simulink model "BEV_Laengsdynamikmodell_v2"  (R2024a)
settings: configuration reference "SharedConfig" (kept outside this file)
values from neighbouring files (symbols this model uses):
  acc_cycle_flag = 0    [simulink_function_handle_v2.m]
  battery = sim_BTMS_interface(battery,config_battery, config_vehicle)    [init_simulation.m]    (also in simulink_function_handle_v2.m = evalin('base', 'battery'))
  config_battery = read_json_config("config/conf_battery.json")    [Sim_v2.m]    (also in init_simulation.m = evalin('base', 'config_battery'); simulink_function_handle_v2.m = cell_loader(config_battery, bat_cell_capacity, bat_celltype )
  config_gearbox = evalin("base", "config_gearbox")    [simulink_function_handle_v2.m]
  config_Inverter = read_json_config("config/conf_Inverter.json")    [Sim_v2.m]
  config_motor = evalin("base","config_motor")    [simulink_function_handle_v2.m]
  config_vehicle = read_json_config(vehicle_config_file)    [Sim_v2.m]    (also in import_dc_cycle.m = evalin('base', 'config_vehicle'); init_simulation.m = evalin('base', 'config_vehicle'); simulink_function_handle_v2.m = evalin('base','config_vehicle'))
  k_FW = 410/(14e3)^2.5    (= 1.76792471652e-08)    [simulink_function_handle_v2.m]
  ModuleType1 = evalin("base","ModuleType1")    [simulink_function_handle_v2.m]
undefined symbols (not defined in the file or in its folder): Analyse, battery_builder_rtmsupport, GB, gcbh, gearbox_map, ModuleAssembly1, motormap
libraries: spsParallelRLCBranchLib x20, nesl_utility x18, GD_Batterymodel_NSGAII_1_lib x12, BatteryProtection x9, spsControlledCurrentSourceLib x8, spsVoltageMeasurementLib x8, fl_lib x7, dspstat3 x4, spsDCVoltageSourceLib x4, spspowerguiLib x4, simulink x3, eePmsmCurrentReferenceGen x2
(part 4 of 5)

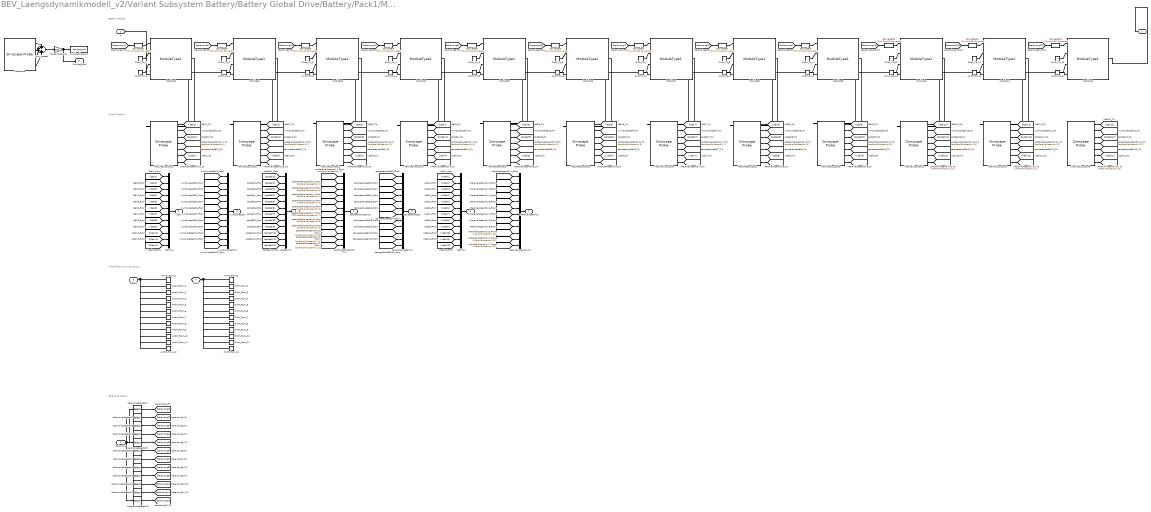
== system BEV_Laengsdynamikmodell_v2/Variant Subsystem Battery/Battery Global Drive/Battery/Pack1/ModuleAssembly1 ==
  note: Battery Modules
  note: Output Signals
  note: Thermal Boundary Conditions
  note: Balancing Signals
  balancing : Inport  PortDimensions=120
  AmbH_From_1 : ConnectionLabel  Label=ambH_1
  AmbH_From_10 : ConnectionLabel  Label=ambH_10
  AmbH_From_11 : ConnectionLabel  Label=ambH_11
  AmbH_From_12 : ConnectionLabel  Label=ambH_12
  AmbH_From_2 : ConnectionLabel  Label=ambH_2
  AmbH_From_3 : ConnectionLabel  Label=ambH_3
  AmbH_From_4 : ConnectionLabel  Label=ambH_4
  AmbH_From_5 : ConnectionLabel  Label=ambH_5
  AmbH_From_6 : ConnectionLabel  Label=ambH_6
  AmbH_From_7 : ConnectionLabel  Label=ambH_7
  AmbH_From_8 : ConnectionLabel  Label=ambH_8
  AmbH_From_9 : ConnectionLabel  Label=ambH_9
  AmbH_To_1 : ConnectionLabel  Label=ambH_1
  AmbH_To_10 : ConnectionLabel  Label=ambH_10
  AmbH_To_11 : ConnectionLabel  Label=ambH_11
  AmbH_To_12 : ConnectionLabel  Label=ambH_12
  AmbH_To_2 : ConnectionLabel  Label=ambH_2
  AmbH_To_3 : ConnectionLabel  Label=ambH_3
  AmbH_To_4 : ConnectionLabel  Label=ambH_4
  AmbH_To_5 : ConnectionLabel  Label=ambH_5
  AmbH_To_6 : ConnectionLabel  Label=ambH_6
  AmbH_To_7 : ConnectionLabel  Label=ambH_7
  AmbH_To_8 : ConnectionLabel  Label=ambH_8
  AmbH_To_9 : ConnectionLabel  Label=ambH_9
  ClntH_From_1 : ConnectionLabel  Label=clntH_1
  ClntH_From_10 : ConnectionLabel  Label=clntH_10
  ClntH_From_11 : ConnectionLabel  Label=clntH_11
  ClntH_From_12 : ConnectionLabel  Label=clntH_12
  ClntH_From_2 : ConnectionLabel  Label=clntH_2
  ClntH_From_3 : ConnectionLabel  Label=clntH_3
  ClntH_From_4 : ConnectionLabel  Label=clntH_4
  ClntH_From_5 : ConnectionLabel  Label=clntH_5
  ClntH_From_6 : ConnectionLabel  Label=clntH_6
  ClntH_From_7 : ConnectionLabel  Label=clntH_7
  ClntH_From_8 : ConnectionLabel  Label=clntH_8
  ClntH_From_9 : ConnectionLabel  Label=clntH_9
  ClntH_To_1 : ConnectionLabel  Label=clntH_1
  ClntH_To_10 : ConnectionLabel  Label=clntH_10
  ClntH_To_11 : ConnectionLabel  Label=clntH_11
  ClntH_To_12 : ConnectionLabel  Label=clntH_12
  ClntH_To_2 : ConnectionLabel  Label=clntH_2
  ClntH_To_3 : ConnectionLabel  Label=clntH_3
  ClntH_To_4 : ConnectionLabel  Label=clntH_4
  ClntH_To_5 : ConnectionLabel  Label=clntH_5
  ClntH_To_6 : ConnectionLabel  Label=clntH_6
  ClntH_To_7 : ConnectionLabel  Label=clntH_7
  ClntH_To_8 : ConnectionLabel  Label=clntH_8
  ClntH_To_9 : ConnectionLabel  Label=clntH_9
  Converter{1..12} (12 alike) : nesl_utility/Simulink-PS Converter  PhysicalDomain=network_engine_domain  SubClassName=ps_input  LeftPortType=input  RightPortType=output  PseudoPeriodic=off  Frequencies=[]  NoiseDistribution=none  NoiseParameters=[]  Unit=1  AffineConversion=off  FilteringAndDerivatives=provide  SimscapeFilterOrder=1  InputFilterTimeConstant=0.001  UdotUserProvided=0
  LossProbe : SimscapeProbe  BoundBlock=59725  Variables={Cell1.power_dissipated, CoolantResistor.Q, balancingResistor.power_dissipated, balancingSwitch.power_dissipated}
  Module01 : GD_Batterymodel_NSGAII_1_lib/Modules/ModuleType1  SOC_vecCell=ModuleType1.SOC_vecCell  T_vecCell=ModuleType1.T_vecCell K  V0_matCell=ModuleType1.V0_matCell V  V_rangeCell=ModuleType1.V_rangeCell V  R0_matCell=ModuleType1.R0_matCell Ohm  AHCell=ModuleType1.AHCell A*hr  extrapolation_optionCell=simscape.enum.extrapolation.nearest  R1_matCell=ModuleType1.R1_matCell Ohm  tau1_matCell=ModuleType1.tau1_matCell s  R2_matCell=ModuleType1.R2_matCell Ohm  tau2_matCell=ModuleType1.tau2_matCell s  thermal_massCell=ModuleType1.thermal_massCell J/K  CoolantResistance=ModuleType1.CoolantResistance K/W  AmbientResistance=ModuleType1.AmbientResistance K/W  CellBalancingClosedResistance=ModuleType1.CellBalancingClosedResistance Ohm  CellBalancingOpenConductance=ModuleType1.CellBalancingOpenConductance 1/Ohm  CellBalancingThreshold=ModuleType1.CellBalancingThreshold  CellBalancingResistance=ModuleType1.CellBalancingResistance Ohm  P=3  S=10  iCell_specify=on  iCell_priority=None  iCell=ModuleAssembly1.Module01.iCell A  iCell_nominal_specify=off  iCell_nominal_unit=A  iCell_nominal_value=1  vCell_specify=on  vCell_priority=None  vCell=ModuleAssembly1.Module01.vCell V  vCell_nominal_specify=off  vCell_nominal_unit=V  vCell_nominal_value=1  socCell_specify=on  socCell_priority=High  socCell=ModuleAssembly1.Module01.socCell  socCell_nominal_specify=off  socCell_nominal_unit=1  socCell_nominal_value=1  numCyclesCell_specify=on  numCyclesCell_priority=High  numCyclesCell=ModuleAssembly1.Module01.numCyclesCell  numCyclesCell_nominal_specify=off  numCyclesCell_nominal_unit=1  numCyclesCell_nominal_value=1  temperatureCell_specify=on  temperatureCell_priority=High  temperatureCell=ModuleAssembly1.Module01.temperatureCell K  temperatureCell_nominal_specify=off  temperatureCell_nominal_unit=K  temperatureCell_nominal_value=1  vParallelAssembly_specify=on  vParallelAssembly_priority=None  vParallelAssembly=ModuleAssembly1.Module01.vParallelAssembly V  vParallelAssembly_nominal_specify=off  vParallelAssembly_nominal_unit=V  vParallelAssembly_nominal_value=1  socParallelAssembly_specify=on  socParallelAssembly_priority=None  socParallelAssembly=ModuleAssembly1.Module01.socParallelAssembly  socParallelAssembly_nominal_specify=off  socParallelAssembly_nominal_unit=1  socParallelAssembly_nominal_value=1
      settings: InternalSimscapePortConfiguration="{\"Bottom\":[{\"id\":\"n\",\"label\":\"-\",\"type\":\"foundation.electrical.electrical\"}],\"Left\":[{\"id\":\"enableCellBalancing\",\"label\":\"CB\",\"type\":\"input\"},{\"id\":\"ClntH\",\"label\":\"CH\",\"type\":\"foundation.thermal.thermal\"},{\"id\":\"AmbH\",\"label\":\"AH\",\"type\":\"foundation.thermal.thermal\"}],\"Right\":[],\"Top\":[{\"id\":\"p\",\"label\":\"+\",\"type\":\"foundation.electrical.electrical\"}]}"
  Module01_outputs : SimscapeProbe  BoundBlock=59725  Variables={iCell, numCyclesCell, socCell, socParallelAssembly, temperatureCell, vCell, vParallelAssembly}
  Module02 : GD_Batterymodel_NSGAII_1_lib/Modules/ModuleType1  SOC_vecCell=ModuleType1.SOC_vecCell  T_vecCell=ModuleType1.T_vecCell K  V0_matCell=ModuleType1.V0_matCell V  V_rangeCell=ModuleType1.V_rangeCell V  R0_matCell=ModuleType1.R0_matCell Ohm  AHCell=ModuleType1.AHCell A*hr  extrapolation_optionCell=simscape.enum.extrapolation.nearest  R1_matCell=ModuleType1.R1_matCell Ohm  tau1_matCell=ModuleType1.tau1_matCell s  R2_matCell=ModuleType1.R2_matCell Ohm  tau2_matCell=ModuleType1.tau2_matCell s  thermal_massCell=ModuleType1.thermal_massCell J/K  CoolantResistance=ModuleType1.CoolantResistance K/W  AmbientResistance=ModuleType1.AmbientResistance K/W  CellBalancingClosedResistance=ModuleType1.CellBalancingClosedResistance Ohm  CellBalancingOpenConductance=ModuleType1.CellBalancingOpenConductance 1/Ohm  CellBalancingThreshold=ModuleType1.CellBalancingThreshold  CellBalancingResistance=ModuleType1.CellBalancingResistance Ohm  P=3  S=10  iCell_specify=on  iCell_priority=None  iCell=ModuleAssembly1.Module02.iCell A  iCell_nominal_specify=off  iCell_nominal_unit=A  iCell_nominal_value=1  vCell_specify=on  vCell_priority=None  vCell=ModuleAssembly1.Module02.vCell V  vCell_nominal_specify=off  vCell_nominal_unit=V  vCell_nominal_value=1  socCell_specify=on  socCell_priority=High  socCell=ModuleAssembly1.Module02.socCell  socCell_nominal_specify=off  socCell_nominal_unit=1  socCell_nominal_value=1  numCyclesCell_specify=on  numCyclesCell_priority=High  numCyclesCell=ModuleAssembly1.Module02.numCyclesCell  numCyclesCell_nominal_specify=off  numCyclesCell_nominal_unit=1  numCyclesCell_nominal_value=1  temperatureCell_specify=on  temperatureCell_priority=High  temperatureCell=ModuleAssembly1.Module02.temperatureCell K  temperatureCell_nominal_specify=off  temperatureCell_nominal_unit=K  temperatureCell_nominal_value=1  vParallelAssembly_specify=on  vParallelAssembly_priority=None  vParallelAssembly=ModuleAssembly1.Module02.vParallelAssembly V  vParallelAssembly_nominal_specify=off  vParallelAssembly_nominal_unit=V  vParallelAssembly_nominal_value=1  socParallelAssembly_specify=on  socParallelAssembly_priority=None  socParallelAssembly=ModuleAssembly1.Module02.socParallelAssembly  socParallelAssembly_nominal_specify=off  socParallelAssembly_nominal_unit=1  socParallelAssembly_nominal_value=1
      settings: InternalSimscapePortConfiguration="{\"Bottom\":[{\"id\":\"n\",\"label\":\"-\",\"type\":\"foundation.electrical.electrical\"}],\"Left\":[{\"id\":\"enableCellBalancing\",\"label\":\"CB\",\"type\":\"input\"},{\"id\":\"ClntH\",\"label\":\"CH\",\"type\":\"foundation.thermal.thermal\"},{\"id\":\"AmbH\",\"label\":\"AH\",\"type\":\"foundation.thermal.thermal\"}],\"Right\":[],\"Top\":[{\"id\":\"p\",\"label\":\"+\",\"type\":\"foundation.electrical.electrical\"}]}"
  Module02_outputs : SimscapeProbe  BoundBlock=59727  Variables={iCell, numCyclesCell, socCell, socParallelAssembly, temperatureCell, vCell, vParallelAssembly}
  Module03 : GD_Batterymodel_NSGAII_1_lib/Modules/ModuleType1  SOC_vecCell=ModuleType1.SOC_vecCell  T_vecCell=ModuleType1.T_vecCell K  V0_matCell=ModuleType1.V0_matCell V  V_rangeCell=ModuleType1.V_rangeCell V  R0_matCell=ModuleType1.R0_matCell Ohm  AHCell=ModuleType1.AHCell A*hr  extrapolation_optionCell=simscape.enum.extrapolation.nearest  R1_matCell=ModuleType1.R1_matCell Ohm  tau1_matCell=ModuleType1.tau1_matCell s  R2_matCell=ModuleType1.R2_matCell Ohm  tau2_matCell=ModuleType1.tau2_matCell s  thermal_massCell=ModuleType1.thermal_massCell J/K  CoolantResistance=ModuleType1.CoolantResistance K/W  AmbientResistance=ModuleType1.AmbientResistance K/W  CellBalancingClosedResistance=ModuleType1.CellBalancingClosedResistance Ohm  CellBalancingOpenConductance=ModuleType1.CellBalancingOpenConductance 1/Ohm  CellBalancingThreshold=ModuleType1.CellBalancingThreshold  CellBalancingResistance=ModuleType1.CellBalancingResistance Ohm  P=3  S=10  iCell_specify=on  iCell_priority=None  iCell=ModuleAssembly1.Module03.iCell A  iCell_nominal_specify=off  iCell_nominal_unit=A  iCell_nominal_value=1  vCell_specify=on  vCell_priority=None  vCell=ModuleAssembly1.Module03.vCell V  vCell_nominal_specify=off  vCell_nominal_unit=V  vCell_nominal_value=1  socCell_specify=on  socCell_priority=High  socCell=ModuleAssembly1.Module03.socCell  socCell_nominal_specify=off  socCell_nominal_unit=1  socCell_nominal_value=1  numCyclesCell_specify=on  numCyclesCell_priority=High  numCyclesCell=ModuleAssembly1.Module03.numCyclesCell  numCyclesCell_nominal_specify=off  numCyclesCell_nominal_unit=1  numCyclesCell_nominal_value=1  temperatureCell_specify=on  temperatureCell_priority=High  temperatureCell=ModuleAssembly1.Module03.temperatureCell K  temperatureCell_nominal_specify=off  temperatureCell_nominal_unit=K  temperatureCell_nominal_value=1  vParallelAssembly_specify=on  vParallelAssembly_priority=None  vParallelAssembly=ModuleAssembly1.Module03.vParallelAssembly V  vParallelAssembly_nominal_specify=off  vParallelAssembly_nominal_unit=V  vParallelAssembly_nominal_value=1  socParallelAssembly_specify=on  socParallelAssembly_priority=None  socParallelAssembly=ModuleAssembly1.Module03.socParallelAssembly  socParallelAssembly_nominal_specify=off  socParallelAssembly_nominal_unit=1  socParallelAssembly_nominal_value=1
      settings: InternalSimscapePortConfiguration="{\"Bottom\":[{\"id\":\"n\",\"label\":\"-\",\"type\":\"foundation.electrical.electrical\"}],\"Left\":[{\"id\":\"enableCellBalancing\",\"label\":\"CB\",\"type\":\"input\"},{\"id\":\"ClntH\",\"label\":\"CH\",\"type\":\"foundation.thermal.thermal\"},{\"id\":\"AmbH\",\"label\":\"AH\",\"type\":\"foundation.thermal.thermal\"}],\"Right\":[],\"Top\":[{\"id\":\"p\",\"label\":\"+\",\"type\":\"foundation.electrical.electrical\"}]}"
  Module03_outputs : SimscapeProbe  BoundBlock=59729  Variables={iCell, numCyclesCell, socCell, socParallelAssembly, temperatureCell, vCell, vParallelAssembly}
  Module04 : GD_Batterymodel_NSGAII_1_lib/Modules/ModuleType1  SOC_vecCell=ModuleType1.SOC_vecCell  T_vecCell=ModuleType1.T_vecCell K  V0_matCell=ModuleType1.V0_matCell V  V_rangeCell=ModuleType1.V_rangeCell V  R0_matCell=ModuleType1.R0_matCell Ohm  AHCell=ModuleType1.AHCell A*hr  extrapolation_optionCell=simscape.enum.extrapolation.nearest  R1_matCell=ModuleType1.R1_matCell Ohm  tau1_matCell=ModuleType1.tau1_matCell s  R2_matCell=ModuleType1.R2_matCell Ohm  tau2_matCell=ModuleType1.tau2_matCell s  thermal_massCell=ModuleType1.thermal_massCell J/K  CoolantResistance=ModuleType1.CoolantResistance K/W  AmbientResistance=ModuleType1.AmbientResistance K/W  CellBalancingClosedResistance=ModuleType1.CellBalancingClosedResistance Ohm  CellBalancingOpenConductance=ModuleType1.CellBalancingOpenConductance 1/Ohm  CellBalancingThreshold=ModuleType1.CellBalancingThreshold  CellBalancingResistance=ModuleType1.CellBalancingResistance Ohm  P=3  S=10  iCell_specify=on  iCell_priority=None  iCell=ModuleAssembly1.Module04.iCell A  iCell_nominal_specify=off  iCell_nominal_unit=A  iCell_nominal_value=1  vCell_specify=on  vCell_priority=None  vCell=ModuleAssembly1.Module04.vCell V  vCell_nominal_specify=off  vCell_nominal_unit=V  vCell_nominal_value=1  socCell_specify=on  socCell_priority=High  socCell=ModuleAssembly1.Module04.socCell  socCell_nominal_specify=off  socCell_nominal_unit=1  socCell_nominal_value=1  numCyclesCell_specify=on  numCyclesCell_priority=High  numCyclesCell=ModuleAssembly1.Module04.numCyclesCell  numCyclesCell_nominal_specify=off  numCyclesCell_nominal_unit=1  numCyclesCell_nominal_value=1  temperatureCell_specify=on  temperatureCell_priority=High  temperatureCell=ModuleAssembly1.Module04.temperatureCell K  temperatureCell_nominal_specify=off  temperatureCell_nominal_unit=K  temperatureCell_nominal_value=1  vParallelAssembly_specify=on  vParallelAssembly_priority=None  vParallelAssembly=ModuleAssembly1.Module04.vParallelAssembly V  vParallelAssembly_nominal_specify=off  vParallelAssembly_nominal_unit=V  vParallelAssembly_nominal_value=1  socParallelAssembly_specify=on  socParallelAssembly_priority=None  socParallelAssembly=ModuleAssembly1.Module04.socParallelAssembly  socParallelAssembly_nominal_specify=off  socParallelAssembly_nominal_unit=1  socParallelAssembly_nominal_value=1
      settings: InternalSimscapePortConfiguration="{\"Bottom\":[{\"id\":\"n\",\"label\":\"-\",\"type\":\"foundation.electrical.electrical\"}],\"Left\":[{\"id\":\"enableCellBalancing\",\"label\":\"CB\",\"type\":\"input\"},{\"id\":\"ClntH\",\"label\":\"CH\",\"type\":\"foundation.thermal.thermal\"},{\"id\":\"AmbH\",\"label\":\"AH\",\"type\":\"foundation.thermal.thermal\"}],\"Right\":[],\"Top\":[{\"id\":\"p\",\"label\":\"+\",\"type\":\"foundation.electrical.electrical\"}]}"
  Module04_outputs : SimscapeProbe  BoundBlock=59731  Variables={iCell, numCyclesCell, socCell, socParallelAssembly, temperatureCell, vCell, vParallelAssembly}
  Module05 : GD_Batterymodel_NSGAII_1_lib/Modules/ModuleType1  SOC_vecCell=ModuleType1.SOC_vecCell  T_vecCell=ModuleType1.T_vecCell K  V0_matCell=ModuleType1.V0_matCell V  V_rangeCell=ModuleType1.V_rangeCell V  R0_matCell=ModuleType1.R0_matCell Ohm  AHCell=ModuleType1.AHCell A*hr  extrapolation_optionCell=simscape.enum.extrapolation.nearest  R1_matCell=ModuleType1.R1_matCell Ohm  tau1_matCell=ModuleType1.tau1_matCell s  R2_matCell=ModuleType1.R2_matCell Ohm  tau2_matCell=ModuleType1.tau2_matCell s  thermal_massCell=ModuleType1.thermal_massCell J/K  CoolantResistance=ModuleType1.CoolantResistance K/W  AmbientResistance=ModuleType1.AmbientResistance K/W  CellBalancingClosedResistance=ModuleType1.CellBalancingClosedResistance Ohm  CellBalancingOpenConductance=ModuleType1.CellBalancingOpenConductance 1/Ohm  CellBalancingThreshold=ModuleType1.CellBalancingThreshold  CellBalancingResistance=ModuleType1.CellBalancingResistance Ohm  P=3  S=10  iCell_specify=on  iCell_priority=None  iCell=ModuleAssembly1.Module05.iCell A  iCell_nominal_specify=off  iCell_nominal_unit=A  iCell_nominal_value=1  vCell_specify=on  vCell_priority=None  vCell=ModuleAssembly1.Module05.vCell V  vCell_nominal_specify=off  vCell_nominal_unit=V  vCell_nominal_value=1  socCell_specify=on  socCell_priority=High  socCell=ModuleAssembly1.Module05.socCell  socCell_nominal_specify=off  socCell_nominal_unit=1  socCell_nominal_value=1  numCyclesCell_specify=on  numCyclesCell_priority=High  numCyclesCell=ModuleAssembly1.Module05.numCyclesCell  numCyclesCell_nominal_specify=off  numCyclesCell_nominal_unit=1  numCyclesCell_nominal_value=1  temperatureCell_specify=on  temperatureCell_priority=High  temperatureCell=ModuleAssembly1.Module05.temperatureCell K  temperatureCell_nominal_specify=off  temperatureCell_nominal_unit=K  temperatureCell_nominal_value=1  vParallelAssembly_specify=on  vParallelAssembly_priority=None  vParallelAssembly=ModuleAssembly1.Module05.vParallelAssembly V  vParallelAssembly_nominal_specify=off  vParallelAssembly_nominal_unit=V  vParallelAssembly_nominal_value=1  socParallelAssembly_specify=on  socParallelAssembly_priority=None  socParallelAssembly=ModuleAssembly1.Module05.socParallelAssembly  socParallelAssembly_nominal_specify=off  socParallelAssembly_nominal_unit=1  socParallelAssembly_nominal_value=1
      settings: InternalSimscapePortConfiguration="{\"Bottom\":[{\"id\":\"n\",\"label\":\"-\",\"type\":\"foundation.electrical.electrical\"}],\"Left\":[{\"id\":\"enableCellBalancing\",\"label\":\"CB\",\"type\":\"input\"},{\"id\":\"ClntH\",\"label\":\"CH\",\"type\":\"foundation.thermal.thermal\"},{\"id\":\"AmbH\",\"label\":\"AH\",\"type\":\"foundation.thermal.thermal\"}],\"Right\":[],\"Top\":[{\"id\":\"p\",\"label\":\"+\",\"type\":\"foundation.electrical.electrical\"}]}"
  Module05_outputs : SimscapeProbe  BoundBlock=59733  Variables={iCell, numCyclesCell, socCell, socParallelAssembly, temperatureCell, vCell, vParallelAssembly}
  Module06 : GD_Batterymodel_NSGAII_1_lib/Modules/ModuleType1  SOC_vecCell=ModuleType1.SOC_vecCell  T_vecCell=ModuleType1.T_vecCell K  V0_matCell=ModuleType1.V0_matCell V  V_rangeCell=ModuleType1.V_rangeCell V  R0_matCell=ModuleType1.R0_matCell Ohm  AHCell=ModuleType1.AHCell A*hr  extrapolation_optionCell=simscape.enum.extrapolation.nearest  R1_matCell=ModuleType1.R1_matCell Ohm  tau1_matCell=ModuleType1.tau1_matCell s  R2_matCell=ModuleType1.R2_matCell Ohm  tau2_matCell=ModuleType1.tau2_matCell s  thermal_massCell=ModuleType1.thermal_massCell J/K  CoolantResistance=ModuleType1.CoolantResistance K/W  AmbientResistance=ModuleType1.AmbientResistance K/W  CellBalancingClosedResistance=ModuleType1.CellBalancingClosedResistance Ohm  CellBalancingOpenConductance=ModuleType1.CellBalancingOpenConductance 1/Ohm  CellBalancingThreshold=ModuleType1.CellBalancingThreshold  CellBalancingResistance=ModuleType1.CellBalancingResistance Ohm  P=3  S=10  iCell_specify=on  iCell_priority=None  iCell=ModuleAssembly1.Module06.iCell A  iCell_nominal_specify=off  iCell_nominal_unit=A  iCell_nominal_value=1  vCell_specify=on  vCell_priority=None  vCell=ModuleAssembly1.Module06.vCell V  vCell_nominal_specify=off  vCell_nominal_unit=V  vCell_nominal_value=1  socCell_specify=on  socCell_priority=High  socCell=ModuleAssembly1.Module06.socCell  socCell_nominal_specify=off  socCell_nominal_unit=1  socCell_nominal_value=1  numCyclesCell_specify=on  numCyclesCell_priority=High  numCyclesCell=ModuleAssembly1.Module06.numCyclesCell  numCyclesCell_nominal_specify=off  numCyclesCell_nominal_unit=1  numCyclesCell_nominal_value=1  temperatureCell_specify=on  temperatureCell_priority=High  temperatureCell=ModuleAssembly1.Module06.temperatureCell K  temperatureCell_nominal_specify=off  temperatureCell_nominal_unit=K  temperatureCell_nominal_value=1  vParallelAssembly_specify=on  vParallelAssembly_priority=None  vParallelAssembly=ModuleAssembly1.Module06.vParallelAssembly V  vParallelAssembly_nominal_specify=off  vParallelAssembly_nominal_unit=V  vParallelAssembly_nominal_value=1  socParallelAssembly_specify=on  socParallelAssembly_priority=None  socParallelAssembly=ModuleAssembly1.Module06.socParallelAssembly  socParallelAssembly_nominal_specify=off  socParallelAssembly_nominal_unit=1  socParallelAssembly_nominal_value=1
      settings: InternalSimscapePortConfiguration="{\"Bottom\":[{\"id\":\"n\",\"label\":\"-\",\"type\":\"foundation.electrical.electrical\"}],\"Left\":[{\"id\":\"enableCellBalancing\",\"label\":\"CB\",\"type\":\"input\"},{\"id\":\"ClntH\",\"label\":\"CH\",\"type\":\"foundation.thermal.thermal\"},{\"id\":\"AmbH\",\"label\":\"AH\",\"type\":\"foundation.thermal.thermal\"}],\"Right\":[],\"Top\":[{\"id\":\"p\",\"label\":\"+\",\"type\":\"foundation.electrical.electrical\"}]}"
  Module06_outputs : SimscapeProbe  BoundBlock=59735  Variables={iCell, numCyclesCell, socCell, socParallelAssembly, temperatureCell, vCell, vParallelAssembly}
  Module07 : GD_Batterymodel_NSGAII_1_lib/Modules/ModuleType1  SOC_vecCell=ModuleType1.SOC_vecCell  T_vecCell=ModuleType1.T_vecCell K  V0_matCell=ModuleType1.V0_matCell V  V_rangeCell=ModuleType1.V_rangeCell V  R0_matCell=ModuleType1.R0_matCell Ohm  AHCell=ModuleType1.AHCell A*hr  extrapolation_optionCell=simscape.enum.extrapolation.nearest  R1_matCell=ModuleType1.R1_matCell Ohm  tau1_matCell=ModuleType1.tau1_matCell s  R2_matCell=ModuleType1.R2_matCell Ohm  tau2_matCell=ModuleType1.tau2_matCell s  thermal_massCell=ModuleType1.thermal_massCell J/K  CoolantResistance=ModuleType1.CoolantResistance K/W  AmbientResistance=ModuleType1.AmbientResistance K/W  CellBalancingClosedResistance=ModuleType1.CellBalancingClosedResistance Ohm  CellBalancingOpenConductance=ModuleType1.CellBalancingOpenConductance 1/Ohm  CellBalancingThreshold=ModuleType1.CellBalancingThreshold  CellBalancingResistance=ModuleType1.CellBalancingResistance Ohm  P=3  S=10  iCell_specify=on  iCell_priority=None  iCell=ModuleAssembly1.Module07.iCell A  iCell_nominal_specify=off  iCell_nominal_unit=A  iCell_nominal_value=1  vCell_specify=on  vCell_priority=None  vCell=ModuleAssembly1.Module07.vCell V  vCell_nominal_specify=off  vCell_nominal_unit=V  vCell_nominal_value=1  socCell_specify=on  socCell_priority=High  socCell=ModuleAssembly1.Module07.socCell  socCell_nominal_specify=off  socCell_nominal_unit=1  socCell_nominal_value=1  numCyclesCell_specify=on  numCyclesCell_priority=High  numCyclesCell=ModuleAssembly1.Module07.numCyclesCell  numCyclesCell_nominal_specify=off  numCyclesCell_nominal_unit=1  numCyclesCell_nominal_value=1  temperatureCell_specify=on  temperatureCell_priority=High  temperatureCell=ModuleAssembly1.Module07.temperatureCell K  temperatureCell_nominal_specify=off  temperatureCell_nominal_unit=K  temperatureCell_nominal_value=1  vParallelAssembly_specify=on  vParallelAssembly_priority=None  vParallelAssembly=ModuleAssembly1.Module07.vParallelAssembly V  vParallelAssembly_nominal_specify=off  vParallelAssembly_nominal_unit=V  vParallelAssembly_nominal_value=1  socParallelAssembly_specify=on  socParallelAssembly_priority=None  socParallelAssembly=ModuleAssembly1.Module07.socParallelAssembly  socParallelAssembly_nominal_specify=off  socParallelAssembly_nominal_unit=1  socParallelAssembly_nominal_value=1
      settings: InternalSimscapePortConfiguration="{\"Bottom\":[{\"id\":\"n\",\"label\":\"-\",\"type\":\"foundation.electrical.electrical\"}],\"Left\":[{\"id\":\"enableCellBalancing\",\"label\":\"CB\",\"type\":\"input\"},{\"id\":\"ClntH\",\"label\":\"CH\",\"type\":\"foundation.thermal.thermal\"},{\"id\":\"AmbH\",\"label\":\"AH\",\"type\":\"foundation.thermal.thermal\"}],\"Right\":[],\"Top\":[{\"id\":\"p\",\"label\":\"+\",\"type\":\"foundation.electrical.electrical\"}]}"
  Module07_outputs : SimscapeProbe  BoundBlock=59737  Variables={iCell, numCyclesCell, socCell, socParallelAssembly, temperatureCell, vCell, vParallelAssembly}
  Module08 : GD_Batterymodel_NSGAII_1_lib/Modules/ModuleType1  SOC_vecCell=ModuleType1.SOC_vecCell  T_vecCell=ModuleType1.T_vecCell K  V0_matCell=ModuleType1.V0_matCell V  V_rangeCell=ModuleType1.V_rangeCell V  R0_matCell=ModuleType1.R0_matCell Ohm  AHCell=ModuleType1.AHCell A*hr  extrapolation_optionCell=simscape.enum.extrapolation.nearest  R1_matCell=ModuleType1.R1_matCell Ohm  tau1_matCell=ModuleType1.tau1_matCell s  R2_matCell=ModuleType1.R2_matCell Ohm  tau2_matCell=ModuleType1.tau2_matCell s  thermal_massCell=ModuleType1.thermal_massCell J/K  CoolantResistance=ModuleType1.CoolantResistance K/W  AmbientResistance=ModuleType1.AmbientResistance K/W  CellBalancingClosedResistance=ModuleType1.CellBalancingClosedResistance Ohm  CellBalancingOpenConductance=ModuleType1.CellBalancingOpenConductance 1/Ohm  CellBalancingThreshold=ModuleType1.CellBalancingThreshold  CellBalancingResistance=ModuleType1.CellBalancingResistance Ohm  P=3  S=10  iCell_specify=on  iCell_priority=None  iCell=ModuleAssembly1.Module08.iCell A  iCell_nominal_specify=off  iCell_nominal_unit=A  iCell_nominal_value=1  vCell_specify=on  vCell_priority=None  vCell=ModuleAssembly1.Module08.vCell V  vCell_nominal_specify=off  vCell_nominal_unit=V  vCell_nominal_value=1  socCell_specify=on  socCell_priority=High  socCell=ModuleAssembly1.Module08.socCell  socCell_nominal_specify=off  socCell_nominal_unit=1  socCell_nominal_value=1  numCyclesCell_specify=on  numCyclesCell_priority=High  numCyclesCell=ModuleAssembly1.Module08.numCyclesCell  numCyclesCell_nominal_specify=off  numCyclesCell_nominal_unit=1  numCyclesCell_nominal_value=1  temperatureCell_specify=on  temperatureCell_priority=High  temperatureCell=ModuleAssembly1.Module08.temperatureCell K  temperatureCell_nominal_specify=off  temperatureCell_nominal_unit=K  temperatureCell_nominal_value=1  vParallelAssembly_specify=on  vParallelAssembly_priority=None  vParallelAssembly=ModuleAssembly1.Module08.vParallelAssembly V  vParallelAssembly_nominal_specify=off  vParallelAssembly_nominal_unit=V  vParallelAssembly_nominal_value=1  socParallelAssembly_specify=on  socParallelAssembly_priority=None  socParallelAssembly=ModuleAssembly1.Module08.socParallelAssembly  socParallelAssembly_nominal_specify=off  socParallelAssembly_nominal_unit=1  socParallelAssembly_nominal_value=1
      settings: InternalSimscapePortConfiguration="{\"Bottom\":[{\"id\":\"n\",\"label\":\"-\",\"type\":\"foundation.electrical.electrical\"}],\"Left\":[{\"id\":\"enableCellBalancing\",\"label\":\"CB\",\"type\":\"input\"},{\"id\":\"ClntH\",\"label\":\"CH\",\"type\":\"foundation.thermal.thermal\"},{\"id\":\"AmbH\",\"label\":\"AH\",\"type\":\"foundation.thermal.thermal\"}],\"Right\":[],\"Top\":[{\"id\":\"p\",\"label\":\"+\",\"type\":\"foundation.electrical.electrical\"}]}"
  Module08_outputs : SimscapeProbe  BoundBlock=59739  Variables={iCell, numCyclesCell, socCell, socParallelAssembly, temperatureCell, vCell, vParallelAssembly}
  Module09 : GD_Batterymodel_NSGAII_1_lib/Modules/ModuleType1  SOC_vecCell=ModuleType1.SOC_vecCell  T_vecCell=ModuleType1.T_vecCell K  V0_matCell=ModuleType1.V0_matCell V  V_rangeCell=ModuleType1.V_rangeCell V  R0_matCell=ModuleType1.R0_matCell Ohm  AHCell=ModuleType1.AHCell A*hr  extrapolation_optionCell=simscape.enum.extrapolation.nearest  R1_matCell=ModuleType1.R1_matCell Ohm  tau1_matCell=ModuleType1.tau1_matCell s  R2_matCell=ModuleType1.R2_matCell Ohm  tau2_matCell=ModuleType1.tau2_matCell s  thermal_massCell=ModuleType1.thermal_massCell J/K  CoolantResistance=ModuleType1.CoolantResistance K/W  AmbientResistance=ModuleType1.AmbientResistance K/W  CellBalancingClosedResistance=ModuleType1.CellBalancingClosedResistance Ohm  CellBalancingOpenConductance=ModuleType1.CellBalancingOpenConductance 1/Ohm  CellBalancingThreshold=ModuleType1.CellBalancingThreshold  CellBalancingResistance=ModuleType1.CellBalancingResistance Ohm  P=3  S=10  iCell_specify=on  iCell_priority=None  iCell=ModuleAssembly1.Module09.iCell A  iCell_nominal_specify=off  iCell_nominal_unit=A  iCell_nominal_value=1  vCell_specify=on  vCell_priority=None  vCell=ModuleAssembly1.Module09.vCell V  vCell_nominal_specify=off  vCell_nominal_unit=V  vCell_nominal_value=1  socCell_specify=on  socCell_priority=High  socCell=ModuleAssembly1.Module09.socCell  socCell_nominal_specify=off  socCell_nominal_unit=1  socCell_nominal_value=1  numCyclesCell_specify=on  numCyclesCell_priority=High  numCyclesCell=ModuleAssembly1.Module09.numCyclesCell  numCyclesCell_nominal_specify=off  numCyclesCell_nominal_unit=1  numCyclesCell_nominal_value=1  temperatureCell_specify=on  temperatureCell_priority=High  temperatureCell=ModuleAssembly1.Module09.temperatureCell K  temperatureCell_nominal_specify=off  temperatureCell_nominal_unit=K  temperatureCell_nominal_value=1  vParallelAssembly_specify=on  vParallelAssembly_priority=None  vParallelAssembly=ModuleAssembly1.Module09.vParallelAssembly V  vParallelAssembly_nominal_specify=off  vParallelAssembly_nominal_unit=V  vParallelAssembly_nominal_value=1  socParallelAssembly_specify=on  socParallelAssembly_priority=None  socParallelAssembly=ModuleAssembly1.Module09.socParallelAssembly  socParallelAssembly_nominal_specify=off  socParallelAssembly_nominal_unit=1  socParallelAssembly_nominal_value=1
      settings: InternalSimscapePortConfiguration="{\"Bottom\":[{\"id\":\"n\",\"label\":\"-\",\"type\":\"foundation.electrical.electrical\"}],\"Left\":[{\"id\":\"enableCellBalancing\",\"label\":\"CB\",\"type\":\"input\"},{\"id\":\"ClntH\",\"label\":\"CH\",\"type\":\"foundation.thermal.thermal\"},{\"id\":\"AmbH\",\"label\":\"AH\",\"type\":\"foundation.thermal.thermal\"}],\"Right\":[],\"Top\":[{\"id\":\"p\",\"label\":\"+\",\"type\":\"foundation.electrical.electrical\"}]}"
  Module09_outputs : SimscapeProbe  BoundBlock=59741  Variables={iCell, numCyclesCell, socCell, socParallelAssembly, temperatureCell, vCell, vParallelAssembly}
  Module10 : GD_Batterymodel_NSGAII_1_lib/Modules/ModuleType1  SOC_vecCell=ModuleType1.SOC_vecCell  T_vecCell=ModuleType1.T_vecCell K  V0_matCell=ModuleType1.V0_matCell V  V_rangeCell=ModuleType1.V_rangeCell V  R0_matCell=ModuleType1.R0_matCell Ohm  AHCell=ModuleType1.AHCell A*hr  extrapolation_optionCell=simscape.enum.extrapolation.nearest  R1_matCell=ModuleType1.R1_matCell Ohm  tau1_matCell=ModuleType1.tau1_matCell s  R2_matCell=ModuleType1.R2_matCell Ohm  tau2_matCell=ModuleType1.tau2_matCell s  thermal_massCell=ModuleType1.thermal_massCell J/K  CoolantResistance=ModuleType1.CoolantResistance K/W  AmbientResistance=ModuleType1.AmbientResistance K/W  CellBalancingClosedResistance=ModuleType1.CellBalancingClosedResistance Ohm  CellBalancingOpenConductance=ModuleType1.CellBalancingOpenConductance 1/Ohm  CellBalancingThreshold=ModuleType1.CellBalancingThreshold  CellBalancingResistance=ModuleType1.CellBalancingResistance Ohm  P=3  S=10  iCell_specify=on  iCell_priority=None  iCell=ModuleAssembly1.Module10.iCell A  iCell_nominal_specify=off  iCell_nominal_unit=A  iCell_nominal_value=1  vCell_specify=on  vCell_priority=None  vCell=ModuleAssembly1.Module10.vCell V  vCell_nominal_specify=off  vCell_nominal_unit=V  vCell_nominal_value=1  socCell_specify=on  socCell_priority=High  socCell=ModuleAssembly1.Module10.socCell  socCell_nominal_specify=off  socCell_nominal_unit=1  socCell_nominal_value=1  numCyclesCell_specify=on  numCyclesCell_priority=High  numCyclesCell=ModuleAssembly1.Module10.numCyclesCell  numCyclesCell_nominal_specify=off  numCyclesCell_nominal_unit=1  numCyclesCell_nominal_value=1  temperatureCell_specify=on  temperatureCell_priority=High  temperatureCell=ModuleAssembly1.Module10.temperatureCell K  temperatureCell_nominal_specify=off  temperatureCell_nominal_unit=K  temperatureCell_nominal_value=1  vParallelAssembly_specify=on  vParallelAssembly_priority=None  vParallelAssembly=ModuleAssembly1.Module10.vParallelAssembly V  vParallelAssembly_nominal_specify=off  vParallelAssembly_nominal_unit=V  vParallelAssembly_nominal_value=1  socParallelAssembly_specify=on  socParallelAssembly_priority=None  socParallelAssembly=ModuleAssembly1.Module10.socParallelAssembly  socParallelAssembly_nominal_specify=off  socParallelAssembly_nominal_unit=1  socParallelAssembly_nominal_value=1
      settings: InternalSimscapePortConfiguration="{\"Bottom\":[{\"id\":\"n\",\"label\":\"-\",\"type\":\"foundation.electrical.electrical\"}],\"Left\":[{\"id\":\"enableCellBalancing\",\"label\":\"CB\",\"type\":\"input\"},{\"id\":\"ClntH\",\"label\":\"CH\",\"type\":\"foundation.thermal.thermal\"},{\"id\":\"AmbH\",\"label\":\"AH\",\"type\":\"foundation.thermal.thermal\"}],\"Right\":[],\"Top\":[{\"id\":\"p\",\"label\":\"+\",\"type\":\"foundation.electrical.electrical\"}]}"
  Module10_outputs : SimscapeProbe  BoundBlock=59743  Variables={iCell, numCyclesCell, socCell, socParallelAssembly, temperatureCell, vCell, vParallelAssembly}
  Module11 : GD_Batterymodel_NSGAII_1_lib/Modules/ModuleType1  SOC_vecCell=ModuleType1.SOC_vecCell  T_vecCell=ModuleType1.T_vecCell K  V0_matCell=ModuleType1.V0_matCell V  V_rangeCell=ModuleType1.V_rangeCell V  R0_matCell=ModuleType1.R0_matCell Ohm  AHCell=ModuleType1.AHCell A*hr  extrapolation_optionCell=simscape.enum.extrapolation.nearest  R1_matCell=ModuleType1.R1_matCell Ohm  tau1_matCell=ModuleType1.tau1_matCell s  R2_matCell=ModuleType1.R2_matCell Ohm  tau2_matCell=ModuleType1.tau2_matCell s  thermal_massCell=ModuleType1.thermal_massCell J/K  CoolantResistance=ModuleType1.CoolantResistance K/W  AmbientResistance=ModuleType1.AmbientResistance K/W  CellBalancingClosedResistance=ModuleType1.CellBalancingClosedResistance Ohm  CellBalancingOpenConductance=ModuleType1.CellBalancingOpenConductance 1/Ohm  CellBalancingThreshold=ModuleType1.CellBalancingThreshold  CellBalancingResistance=ModuleType1.CellBalancingResistance Ohm  P=3  S=10  iCell_specify=on  iCell_priority=None  iCell=ModuleAssembly1.Module11.iCell A  iCell_nominal_specify=off  iCell_nominal_unit=A  iCell_nominal_value=1  vCell_specify=on  vCell_priority=None  vCell=ModuleAssembly1.Module11.vCell V  vCell_nominal_specify=off  vCell_nominal_unit=V  vCell_nominal_value=1  socCell_specify=on  socCell_priority=High  socCell=ModuleAssembly1.Module11.socCell  socCell_nominal_specify=off  socCell_nominal_unit=1  socCell_nominal_value=1  numCyclesCell_specify=on  numCyclesCell_priority=High  numCyclesCell=ModuleAssembly1.Module11.numCyclesCell  numCyclesCell_nominal_specify=off  numCyclesCell_nominal_unit=1  numCyclesCell_nominal_value=1  temperatureCell_specify=on  temperatureCell_priority=High  temperatureCell=ModuleAssembly1.Module11.temperatureCell K  temperatureCell_nominal_specify=off  temperatureCell_nominal_unit=K  temperatureCell_nominal_value=1  vParallelAssembly_specify=on  vParallelAssembly_priority=None  vParallelAssembly=ModuleAssembly1.Module11.vParallelAssembly V  vParallelAssembly_nominal_specify=off  vParallelAssembly_nominal_unit=V  vParallelAssembly_nominal_value=1  socParallelAssembly_specify=on  socParallelAssembly_priority=None  socParallelAssembly=ModuleAssembly1.Module11.socParallelAssembly  socParallelAssembly_nominal_specify=off  socParallelAssembly_nominal_unit=1  socParallelAssembly_nominal_value=1
      settings: InternalSimscapePortConfiguration="{\"Bottom\":[{\"id\":\"n\",\"label\":\"-\",\"type\":\"foundation.electrical.electrical\"}],\"Left\":[{\"id\":\"enableCellBalancing\",\"label\":\"CB\",\"type\":\"input\"},{\"id\":\"ClntH\",\"label\":\"CH\",\"type\":\"foundation.thermal.thermal\"},{\"id\":\"AmbH\",\"label\":\"AH\",\"type\":\"foundation.thermal.thermal\"}],\"Right\":[],\"Top\":[{\"id\":\"p\",\"label\":\"+\",\"type\":\"foundation.electrical.electrical\"}]}"
  Module11_outputs : SimscapeProbe  BoundBlock=59745  Variables={iCell, numCyclesCell, socCell, socParallelAssembly, temperatureCell, vCell, vParallelAssembly}
  Module12 : GD_Batterymodel_NSGAII_1_lib/Modules/ModuleType1  SOC_vecCell=ModuleType1.SOC_vecCell  T_vecCell=ModuleType1.T_vecCell K  V0_matCell=ModuleType1.V0_matCell V  V_rangeCell=ModuleType1.V_rangeCell V  R0_matCell=ModuleType1.R0_matCell Ohm  AHCell=ModuleType1.AHCell A*hr  extrapolation_optionCell=simscape.enum.extrapolation.nearest  R1_matCell=ModuleType1.R1_matCell Ohm  tau1_matCell=ModuleType1.tau1_matCell s  R2_matCell=ModuleType1.R2_matCell Ohm  tau2_matCell=ModuleType1.tau2_matCell s  thermal_massCell=ModuleType1.thermal_massCell J/K  CoolantResistance=ModuleType1.CoolantResistance K/W  AmbientResistance=ModuleType1.AmbientResistance K/W  CellBalancingClosedResistance=ModuleType1.CellBalancingClosedResistance Ohm  CellBalancingOpenConductance=ModuleType1.CellBalancingOpenConductance 1/Ohm  CellBalancingThreshold=ModuleType1.CellBalancingThreshold  CellBalancingResistance=ModuleType1.CellBalancingResistance Ohm  P=3  S=10  iCell_specify=on  iCell_priority=None  iCell=ModuleAssembly1.Module12.iCell A  iCell_nominal_specify=off  iCell_nominal_unit=A  iCell_nominal_value=1  vCell_specify=on  vCell_priority=None  vCell=ModuleAssembly1.Module12.vCell V  vCell_nominal_specify=off  vCell_nominal_unit=V  vCell_nominal_value=1  socCell_specify=on  socCell_priority=High  socCell=ModuleAssembly1.Module12.socCell  socCell_nominal_specify=off  socCell_nominal_unit=1  socCell_nominal_value=1  numCyclesCell_specify=on  numCyclesCell_priority=High  numCyclesCell=ModuleAssembly1.Module12.numCyclesCell  numCyclesCell_nominal_specify=off  numCyclesCell_nominal_unit=1  numCyclesCell_nominal_value=1  temperatureCell_specify=on  temperatureCell_priority=High  temperatureCell=ModuleAssembly1.Module12.temperatureCell K  temperatureCell_nominal_specify=off  temperatureCell_nominal_unit=K  temperatureCell_nominal_value=1  vParallelAssembly_specify=on  vParallelAssembly_priority=None  vParallelAssembly=ModuleAssembly1.Module12.vParallelAssembly V  vParallelAssembly_nominal_specify=off  vParallelAssembly_nominal_unit=V  vParallelAssembly_nominal_value=1  socParallelAssembly_specify=on  socParallelAssembly_priority=None  socParallelAssembly=ModuleAssembly1.Module12.socParallelAssembly  socParallelAssembly_nominal_specify=off  socParallelAssembly_nominal_unit=1  socParallelAssembly_nominal_value=1
      settings: InternalSimscapePortConfiguration="{\"Bottom\":[{\"id\":\"n\",\"label\":\"-\",\"type\":\"foundation.electrical.electrical\"}],\"Left\":[{\"id\":\"enableCellBalancing\",\"label\":\"CB\",\"type\":\"input\"},{\"id\":\"ClntH\",\"label\":\"CH\",\"type\":\"foundation.thermal.thermal\"},{\"id\":\"AmbH\",\"label\":\"AH\",\"type\":\"foundation.thermal.thermal\"}],\"Right\":[],\"Top\":[{\"id\":\"p\",\"label\":\"+\",\"type\":\"foundation.electrical.electrical\"}]}"
  Module12_outputs : SimscapeProbe  BoundBlock=59747  Variables={iCell, numCyclesCell, socCell, socParallelAssembly, temperatureCell, vCell, vParallelAssembly}
  Scale_TotalLoss : Gain  Gain=360
  Sum_Losses : Sum  Inputs=++++
  balancingSelector1 : Selector  InputPortWidth=120  IndexOptions=Index vector (dialog)  Indices="[1   2   3   4   5   6   7   8   9  10]"  OutputSizes=1
  balancingSelector10 : Selector  InputPortWidth=120  IndexOptions=Index vector (dialog)  Indices="[91   92   93   94   95   96   97   98   99  100]"  OutputSizes=1
  balancingSelector11 : Selector  InputPortWidth=120  IndexOptions=Index vector (dialog)  Indices="[101  102  103  104  105  106  107  108  109  110]"  OutputSizes=1
  balancingSelector12 : Selector  InputPortWidth=120  IndexOptions=Index vector (dialog)  Indices="[111  112  113  114  115  116  117  118  119  120]"  OutputSizes=1
  balancingSelector2 : Selector  InputPortWidth=120  IndexOptions=Index vector (dialog)  Indices="[11  12  13  14  15  16  17  18  19  20]"  OutputSizes=1
  balancingSelector3 : Selector  InputPortWidth=120  IndexOptions=Index vector (dialog)  Indices="[21  22  23  24  25  26  27  28  29  30]"  OutputSizes=1
  balancingSelector4 : Selector  InputPortWidth=120  IndexOptions=Index vector (dialog)  Indices="[31  32  33  34  35  36  37  38  39  40]"  OutputSizes=1
  balancingSelector5 : Selector  InputPortWidth=120  IndexOptions=Index vector (dialog)  Indices="[41  42  43  44  45  46  47  48  49  50]"  OutputSizes=1
  balancingSelector6 : Selector  InputPortWidth=120  IndexOptions=Index vector (dialog)  Indices="[51  52  53  54  55  56  57  58  59  60]"  OutputSizes=1
  balancingSelector7 : Selector  InputPortWidth=120  IndexOptions=Index vector (dialog)  Indices="[61  62  63  64  65  66  67  68  69  70]"  OutputSizes=1
  balancingSelector8 : Selector  InputPortWidth=120  IndexOptions=Index vector (dialog)  Indices="[71  72  73  74  75  76  77  78  79  80]"  OutputSizes=1
  balancingSelector9 : Selector  InputPortWidth=120  IndexOptions=Index vector (dialog)  Indices="[81  82  83  84  85  86  87  88  89  90]"  OutputSizes=1
  iCellMux : Mux  Inputs=12
  numCyclesCellMux : Mux  Inputs=12
  sink_bat_loss_out : ToWorkspace  VariableName=bat_loss_out  SaveFormat=Timeseries  SampleTime=-1
  socCellMux : Mux  Inputs=12
  socParallelAssemblyMux : Mux  Inputs=12
  temperatureCellMux : Mux  Inputs=12
  vCellMux : Mux  Inputs=12
  vParallelAssemblyMux : Mux  Inputs=12
  + : PMIOPort  Side=Left
  - : PMIOPort  Port=2  Side=Right
  AmbH : PMIOPort  Port=3  Side=Right  ConnectionType=Connection: foundation.thermal.thermal
  ClntH : PMIOPort  Port=4  Side=Right  ConnectionType=Connection: foundation.thermal.thermal
  iCell : Outport
  numCyclesCell : Outport  Port=2
  socCell : Outport  Port=3
  socParallelAssembly : Outport  Port=4
  temperatureCell : Outport  Port=5
  vCell : Outport  Port=6
  vParallelAssembly : Outport  Port=7
  Out_bat_loss : Outport  Port=8
  wires:
  Module01_outputs/1 -> [iCell1]
  iCellMux/1 -> iCell/1
  [iCell1] -> iCellMux/1
  Module01_outputs/2 -> [numCyclesCell1]
  numCyclesCellMux/1 -> numCyclesCell/1
  [numCyclesCell1] -> numCyclesCellMux/1
  Module01_outputs/3 -> [socCell1]
  socCellMux/1 -> socCell/1
  [socCell1] -> socCellMux/1
  Module01_outputs/4 -> [socParallelAssembly1]
  socParallelAssemblyMux/1 -> socParallelAssembly/1
  [socParallelAssembly1] -> socParallelAssemblyMux/1
  Module01_outputs/5 -> [temperatureCell1]
  temperatureCellMux/1 -> temperatureCell/1
  [temperatureCell1] -> temperatureCellMux/1
  Module01_outputs/6 -> [vCell1]
  vCellMux/1 -> vCell/1
  [vCell1] -> vCellMux/1
  Module01_outputs/7 -> [vParallelAssembly1]
  vParallelAssemblyMux/1 -> vParallelAssembly/1
  [vParallelAssembly1] -> vParallelAssemblyMux/1
  Module02_outputs/1 -> [iCell2]
  [iCell2] -> iCellMux/2
  Module02_outputs/2 -> [numCyclesCell2]
  [numCyclesCell2] -> numCyclesCellMux/2
  Module02_outputs/3 -> [socCell2]
  [socCell2] -> socCellMux/2
  Module02_outputs/4 -> [socParallelAssembly2]
  [socParallelAssembly2] -> socParallelAssemblyMux/2
  Module02_outputs/5 -> [temperatureCell2]
  [temperatureCell2] -> temperatureCellMux/2
  Module02_outputs/6 -> [vCell2]
  [vCell2] -> vCellMux/2
  Module02_outputs/7 -> [vParallelAssembly2]
  [vParallelAssembly2] -> vParallelAssemblyMux/2
  Module03_outputs/1 -> [iCell3]
  [iCell3] -> iCellMux/3
  Module03_outputs/2 -> [numCyclesCell3]
  [numCyclesCell3] -> numCyclesCellMux/3
  Module03_outputs/3 -> [socCell3]
  [socCell3] -> socCellMux/3
  Module03_outputs/4 -> [socParallelAssembly3]
  [socParallelAssembly3] -> socParallelAssemblyMux/3
  Module03_outputs/5 -> [temperatureCell3]
  [temperatureCell3] -> temperatureCellMux/3
  Module03_outputs/6 -> [vCell3]
  [vCell3] -> vCellMux/3
  Module03_outputs/7 -> [vParallelAssembly3]
  [vParallelAssembly3] -> vParallelAssemblyMux/3
  Module04_outputs/1 -> [iCell4]
  [iCell4] -> iCellMux/4
  Module04_outputs/2 -> [numCyclesCell4]
  [numCyclesCell4] -> numCyclesCellMux/4
  Module04_outputs/3 -> [socCell4]
  [socCell4] -> socCellMux/4
  Module04_outputs/4 -> [socParallelAssembly4]
  [socParallelAssembly4] -> socParallelAssemblyMux/4
  Module04_outputs/5 -> [temperatureCell4]
  [temperatureCell4] -> temperatureCellMux/4
  Module04_outputs/6 -> [vCell4]
  [vCell4] -> vCellMux/4
  Module04_outputs/7 -> [vParallelAssembly4]
  [vParallelAssembly4] -> vParallelAssemblyMux/4
  Module05_outputs/1 -> [iCell5]
  [iCell5] -> iCellMux/5
  Module05_outputs/2 -> [numCyclesCell5]
  [numCyclesCell5] -> numCyclesCellMux/5
  Module05_outputs/3 -> [socCell5]
  [socCell5] -> socCellMux/5
  Module05_outputs/4 -> [socParallelAssembly5]
  [socParallelAssembly5] -> socParallelAssemblyMux/5
  Module05_outputs/5 -> [temperatureCell5]
  [temperatureCell5] -> temperatureCellMux/5
  Module05_outputs/6 -> [vCell5]
  [vCell5] -> vCellMux/5
  Module05_outputs/7 -> [vParallelAssembly5]
  [vParallelAssembly5] -> vParallelAssemblyMux/5
  Module06_outputs/1 -> [iCell6]
  [iCell6] -> iCellMux/6
  Module06_outputs/2 -> [numCyclesCell6]
  [numCyclesCell6] -> numCyclesCellMux/6
  Module06_outputs/3 -> [socCell6]
  [socCell6] -> socCellMux/6
  Module06_outputs/4 -> [socParallelAssembly6]
  [socParallelAssembly6] -> socParallelAssemblyMux/6
  Module06_outputs/5 -> [temperatureCell6]
  [temperatureCell6] -> temperatureCellMux/6
  Module06_outputs/6 -> [vCell6]
  [vCell6] -> vCellMux/6
  Module06_outputs/7 -> [vParallelAssembly6]
  [vParallelAssembly6] -> vParallelAssemblyMux/6
  Module07_outputs/1 -> [iCell7]
  [iCell7] -> iCellMux/7
  Module07_outputs/2 -> [numCyclesCell7]
  [numCyclesCell7] -> numCyclesCellMux/7
  Module07_outputs/3 -> [socCell7]
  [socCell7] -> socCellMux/7
  Module07_outputs/4 -> [socParallelAssembly7]
  [socParallelAssembly7] -> socParallelAssemblyMux/7
  Module07_outputs/5 -> [temperatureCell7]
  [temperatureCell7] -> temperatureCellMux/7
  Module07_outputs/6 -> [vCell7]
  [vCell7] -> vCellMux/7
  Module07_outputs/7 -> [vParallelAssembly7]
  [vParallelAssembly7] -> vParallelAssemblyMux/7
  Module08_outputs/1 -> [iCell8]
  [iCell8] -> iCellMux/8
  Module08_outputs/2 -> [numCyclesCell8]
  [numCyclesCell8] -> numCyclesCellMux/8
  Module08_outputs/3 -> [socCell8]
  [socCell8] -> socCellMux/8
  Module08_outputs/4 -> [socParallelAssembly8]
  [socParallelAssembly8] -> socParallelAssemblyMux/8
  Module08_outputs/5 -> [temperatureCell8]
  [temperatureCell8] -> temperatureCellMux/8
  Module08_outputs/6 -> [vCell8]
  [vCell8] -> vCellMux/8
  Module08_outputs/7 -> [vParallelAssembly8]
  [vParallelAssembly8] -> vParallelAssemblyMux/8
  Module09_outputs/1 -> [iCell9]
  [iCell9] -> iCellMux/9
  Module09_outputs/2 -> [numCyclesCell9]
  [numCyclesCell9] -> numCyclesCellMux/9
  Module09_outputs/3 -> [socCell9]
  [socCell9] -> socCellMux/9
  Module09_outputs/4 -> [socParallelAssembly9]
  [socParallelAssembly9] -> socParallelAssemblyMux/9
  Module09_outputs/5 -> [temperatureCell9]
  [temperatureCell9] -> temperatureCellMux/9
  Module09_outputs/6 -> [vCell9]
  [vCell9] -> vCellMux/9
  Module09_outputs/7 -> [vParallelAssembly9]
  [vParallelAssembly9] -> vParallelAssemblyMux/9
  Module10_outputs/1 -> [iCell10]
  [iCell10] -> iCellMux/10
  Module10_outputs/2 -> [numCyclesCell10]
  [numCyclesCell10] -> numCyclesCellMux/10
  Module10_outputs/3 -> [socCell10]
  [socCell10] -> socCellMux/10
  Module10_outputs/4 -> [socParallelAssembly10]
  [socParallelAssembly10] -> socParallelAssemblyMux/10
  Module10_outputs/5 -> [temperatureCell10]
  [temperatureCell10] -> temperatureCellMux/10
  Module10_outputs/6 -> [vCell10]
  [vCell10] -> vCellMux/10
  Module10_outputs/7 -> [vParallelAssembly10]
  [vParallelAssembly10] -> vParallelAssemblyMux/10
  Module11_outputs/1 -> [iCell11]
  [iCell11] -> iCellMux/11
  Module11_outputs/2 -> [numCyclesCell11]
  [numCyclesCell11] -> numCyclesCellMux/11
  Module11_outputs/3 -> [socCell11]
  [socCell11] -> socCellMux/11
  Module11_outputs/4 -> [socParallelAssembly11]
  [socParallelAssembly11] -> socParallelAssemblyMux/11
  Module11_outputs/5 -> [temperatureCell11]
  [temperatureCell11] -> temperatureCellMux/11
  Module11_outputs/6 -> [vCell11]
  [vCell11] -> vCellMux/11
  Module11_outputs/7 -> [vParallelAssembly11]
  [vParallelAssembly11] -> vParallelAssemblyMux/11
  Module12_outputs/1 -> [iCell12]
  [iCell12] -> iCellMux/12
  Module12_outputs/2 -> [numCyclesCell12]
  [numCyclesCell12] -> numCyclesCellMux/12
  Module12_outputs/3 -> [socCell12]
  [socCell12] -> socCellMux/12
  Module12_outputs/4 -> [socParallelAssembly12]
  [socParallelAssembly12] -> socParallelAssemblyMux/12
  Module12_outputs/5 -> [temperatureCell12]
  [temperatureCell12] -> temperatureCellMux/12
  Module12_outputs/6 -> [vCell12]
  [vCell12] -> vCellMux/12
  Module12_outputs/7 -> [vParallelAssembly12]
  [vParallelAssembly12] -> vParallelAssemblyMux/12
  [balancing1] -> Converter1/1
  balancing/1 -> balancingSelector1/1, balancingSelector2/1, balancingSelector3/1, balancingSelector4/1, balancingSelector5/1, balancingSelector6/1, balancingSelector7/1, balancingSelector8/1, balancingSelector9/1, balancingSelector10/1, balancingSelector11/1, balancingSelector12/1
  balancingSelector1/1 -> [balancing1]
  [balancing2] -> Converter2/1
  balancingSelector2/1 -> [balancing2]
  [balancing3] -> Converter3/1
  balancingSelector3/1 -> [balancing3]
  [balancing4] -> Converter4/1
  balancingSelector4/1 -> [balancing4]
  [balancing5] -> Converter5/1
  balancingSelector5/1 -> [balancing5]
  [balancing6] -> Converter6/1
  balancingSelector6/1 -> [balancing6]
  [balancing7] -> Converter7/1
  balancingSelector7/1 -> [balancing7]
  [balancing8] -> Converter8/1
  balancingSelector8/1 -> [balancing8]
  [balancing9] -> Converter9/1
  balancingSelector9/1 -> [balancing9]
  [balancing10] -> Converter10/1
  balancingSelector10/1 -> [balancing10]
  [balancing11] -> Converter11/1
  balancingSelector11/1 -> [balancing11]
  [balancing12] -> Converter12/1
  balancingSelector12/1 -> [balancing12]
  LossProbe/1 -> Sum_Losses/1
  LossProbe/2 -> Sum_Losses/2
  LossProbe/3 -> Sum_Losses/3
  LossProbe/4 -> Sum_Losses/4
  Sum_Losses/1 -> Scale_TotalLoss/1
  Scale_TotalLoss/1 -> sink_bat_loss_out/1, Out_bat_loss/1
  connections:
  Module02/LConn4 -- Module01/RConn1
  Module03/LConn4 -- Module02/RConn1
  Module04/LConn4 -- Module03/RConn1
  Module05/LConn4 -- Module04/RConn1
  Module06/LConn4 -- Module05/RConn1
  Module07/LConn4 -- Module06/RConn1
  Module08/LConn4 -- Module07/RConn1
  Module09/LConn4 -- Module08/RConn1
  Module10/LConn4 -- Module09/RConn1
  Module11/LConn4 -- Module10/RConn1
  Module12/LConn4 -- Module11/RConn1
  Module01/LConn4 -- +/RConn1
  Module12/RConn1 -- -/RConn1
  AmbH_To_1/LConn1 -- Module01/LConn3
  AmbH_From_1/LConn1 -- AmbH_From_2/LConn1 -- AmbH_From_3/LConn1 -- AmbH_From_4/LConn1 -- AmbH_From_5/LConn1 -- AmbH_From_6/LConn1 -- AmbH_From_7/LConn1 -- AmbH_From_8/LConn1 -- AmbH_From_9/LConn1 -- AmbH_From_10/LConn1 -- AmbH_From_11/LConn1 -- AmbH/RConn1 -- AmbH_From_12/LConn1
  AmbH_To_2/LConn1 -- Module02/LConn3
  AmbH_To_3/LConn1 -- Module03/LConn3
  AmbH_To_4/LConn1 -- Module04/LConn3
  AmbH_To_5/LConn1 -- Module05/LConn3
  AmbH_To_6/LConn1 -- Module06/LConn3
  AmbH_To_7/LConn1 -- Module07/LConn3
  AmbH_To_8/LConn1 -- Module08/LConn3
  AmbH_To_9/LConn1 -- Module09/LConn3
  AmbH_To_10/LConn1 -- Module10/LConn3
  AmbH_To_11/LConn1 -- Module11/LConn3
  AmbH_To_12/LConn1 -- Module12/LConn3
  ClntH_To_1/LConn1 -- Module01/LConn2
  ClntH_From_1/LConn1 -- ClntH_From_2/LConn1 -- ClntH_From_3/LConn1 -- ClntH_From_4/LConn1 -- ClntH_From_5/LConn1 -- ClntH_From_6/LConn1 -- ClntH_From_7/LConn1 -- ClntH_From_8/LConn1 -- ClntH_From_9/LConn1 -- ClntH_From_10/LConn1 -- ClntH_From_11/LConn1 -- ClntH/RConn1 -- ClntH_From_12/LConn1
  ClntH_To_2/LConn1 -- Module02/LConn2
  ClntH_To_3/LConn1 -- Module03/LConn2
  ClntH_To_4/LConn1 -- Module04/LConn2
  ClntH_To_5/LConn1 -- Module05/LConn2
  ClntH_To_6/LConn1 -- Module06/LConn2
  ClntH_To_7/LConn1 -- Module07/LConn2
  ClntH_To_8/LConn1 -- Module08/LConn2
  ClntH_To_9/LConn1 -- Module09/LConn2
  ClntH_To_10/LConn1 -- Module10/LConn2
  ClntH_To_11/LConn1 -- Module11/LConn2
  ClntH_To_12/LConn1 -- Module12/LConn2
  Converter1/RConn1 -- Module01/LConn1
  Converter2/RConn1 -- Module02/LConn1
  Converter3/RConn1 -- Module03/LConn1
  Converter4/RConn1 -- Module04/LConn1
  Converter5/RConn1 -- Module05/LConn1
  Converter6/RConn1 -- Module06/LConn1
  Converter7/RConn1 -- Module07/LConn1
  Converter8/RConn1 -- Module08/LConn1
  Converter9/RConn1 -- Module09/LConn1
  Converter10/RConn1 -- Module10/LConn1
  Converter11/RConn1 -- Module11/LConn1
  Converter12/RConn1 -- Module12/LConn1
